simulink model "Deployment_eject"  (R2018b)
settings: Solver=VariableStepAuto  StartTime=0.0  StopTime=10.0  RelTol=1e-3
settings Model: Creator=Daniel  LastModifiedBy=Daniel

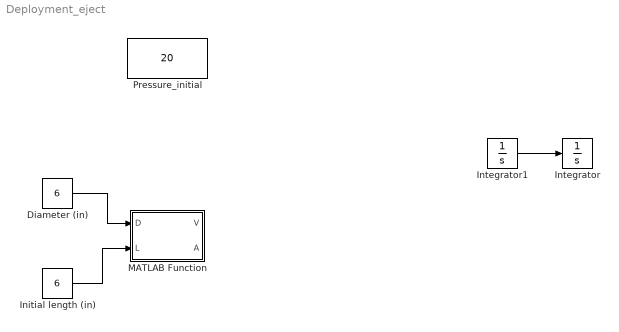
== system Deployment_eject ==
  Diameter (in) : Constant  Value=6
  Initial length (in) : Constant  Value=6
  Integrator : Integrator  InitialCondition=6
  Integrator1 : Integrator  InitialCondition=6
  MATLAB Function : MATLAB Function  TreatAsAtomicUnit=on
  Pressure_initial : Constant  Value=20
  wires:
  Diameter (in)/1 -> MATLAB Function/1(D)
  Initial length (in)/1 -> MATLAB Function/2(L)
  Integrator1/1 -> Integrator/1

== matlab function Deployment_eject/MATLAB Function ==
  data: D input; V output; L input; A output
function [V, A] = volume(D, L)
A = (pi / 4) * D.^2;
V = A * L;
end
